simulink model "S12_Frozen_Radiation_Adapter_v12"  (R2026a)
settings: Solver=FixedStepDiscrete  StopTime=90  FixedStep=0.02
undefined symbols (not defined in the file): s12_v12_model_radiation_step
settings Model: Creator=Jovi  LastModifiedBy=Jovi

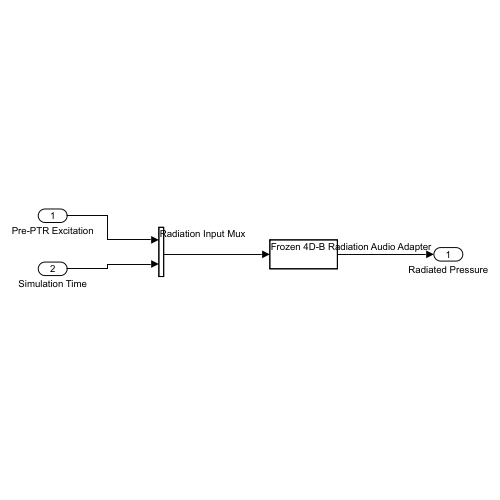
[thumbnail: Simulink's stored preview of the top-level diagram]
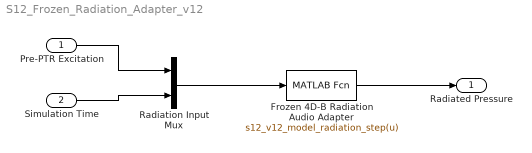
== system S12_Frozen_Radiation_Adapter_v12 ==
  Pre-PTR Excitation : Inport  PortDimensions=960
  Simulation Time : Inport  Port=2  PortDimensions=1
  Frozen 4D-B Radiation Audio Adapter : MATLABFcn  MATLABFcn=s12_v12_model_radiation_step(u)  Output1D=off
  Radiation Input Mux : Mux  Inputs=2
  Radiated Pressure : Outport  PortDimensions=960
  wires:
  Frozen 4D-B Radiation Audio Adapter/1 -> Radiated Pressure/1
  Radiation Input Mux/1 -> Frozen 4D-B Radiation Audio Adapter/1
  Simulation Time/1 -> Radiation Input Mux/2
  Pre-PTR Excitation/1 -> Radiation Input Mux/1
